simulink model "sampleModel334"  (R2021b)
settings: Solver=VariableStepAuto  StartTime=0.0  StopTime=10.0  RelTol=1e-3
undefined symbols (not defined in the file or in its folder): Newton, Raphson
libraries: simulink x13, slpidlib x2
settings Model: Creator=user  LastModifiedBy=user

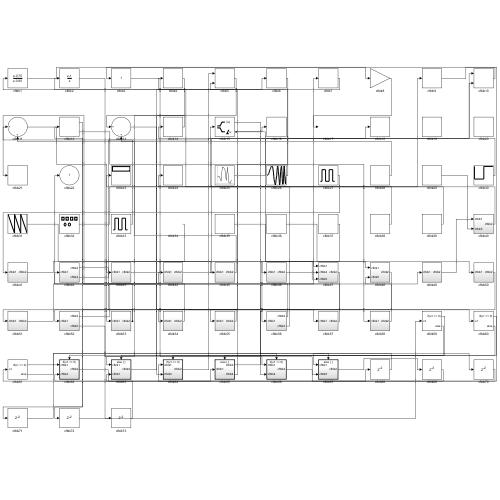
[thumbnail: Simulink's stored preview of the top-level diagram]
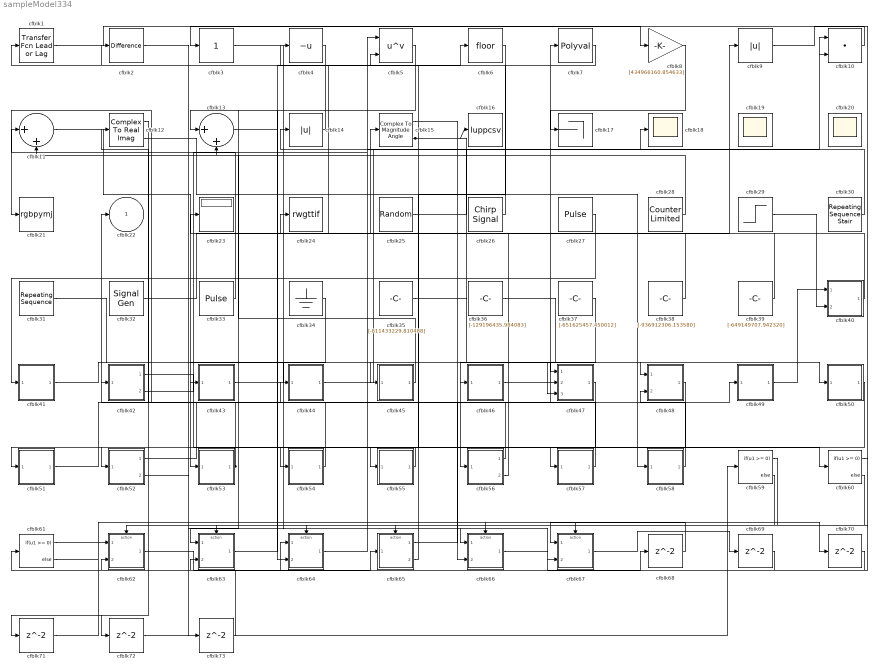
== system sampleModel334 ==
  cfblk1 : simulink/Discrete/Transfer Fcn Lead or Lag  PoleZ=0.95  ZeroZ=0.75  ICPrevOutput=0.0  ICPrevInput=0.0  DoSatur=off
      settings: SourceProductBaseCode=SL
  cfblk10 : DotProduct  InputSameDT=on  OutDataTypeStr=Inherit: Inherit via internal rule
  cfblk11 : Sum  Inputs=|++
  cfblk12 : ComplexToRealImag
  cfblk13 : Sum  Inputs=|++
  cfblk14 : Abs
  cfblk15 : ComplexToMagnitudeAngle
  cfblk16 : ToWorkspace  VariableName=luppcsv  SaveFormat=Timeseries  SampleTime=-1
  cfblk17 : Terminator
  cfblk18 : Scope
  cfblk19 : Scope
      settings: Floating=on
  cfblk2 : simulink/Discrete/Difference  ICPrevInput=0.0  OutMin=[]  OutMax=[]  OutDataTypeStr=Inherit: Inherit via back propagation  OutDataType=fixdt(1, 16)  OutScaling=2^-10  DoSatur=off
  cfblk20 : Scope
      settings: Floating=on
  cfblk21 : ToWorkspace  VariableName=rgbpymj  SaveFormat=Timeseries  SampleTime=-1
  cfblk23 : Display
  cfblk24 : ToWorkspace  VariableName=rwgttif  SaveFormat=Timeseries  SampleTime=-1
  cfblk25 : RandomNumber  Mean=[-31709.471709]  Variance=[21880.294975]  Seed=[988417570.000000]  SampleTime=0.1
  cfblk26 : simulink/Sources/Chirp Signal  f1=[-190654056.309968]  T=[-437298929.840146]  f2=[-613895744.060993]
  cfblk27 : DiscretePulseGenerator  PulseType=Time based  Amplitude=[95953160.588672]  Period=[92796952.421330]  PulseWidth=5  PhaseDelay=[6.000000]
  cfblk28 : simulink/Sources/Counter Limited  uplimit=[666.000000]  tsamp=-1
  cfblk29 : Step  Time=[43.000000]  Before=[594714500.417629]  After=[-95569825.791447]  SampleTime=0
  cfblk3 : simulink/Math Operations/Slider Gain  gain=1  low=0  high=2
  cfblk30 : simulink/Sources/Repeating Sequence Stair  OutValues=[445695939.025532, 871780423.496067]  tsamp=-1  OutMin=[]  OutMax=[]  OutDataTypeStr=double  OutputDataTypeScalingMode=double  OutDataType=fixdt(0,8)  ConRadixGroup=Best Precision: Vector-wise  OutScaling=2^-12
  cfblk31 : simulink/Sources/Repeating Sequence  rep_seq_t=[0 2]  rep_seq_y=[950228293.664763, -742331251.435693]
  cfblk32 : SignalGenerator  WaveForm=square  Amplitude=[-929706620.397252]
  cfblk33 : DiscretePulseGenerator  PulseType=Time based  Amplitude=[171272689.061584]  Period=[21777336.643876]  PulseWidth=5  PhaseDelay=[4.000000]
  cfblk34 : Ground
  cfblk35 : Constant  Value=[-811433229.810488]  SampleTime=1
  cfblk36 : Constant  Value=[-129196435.984083]  SampleTime=1
  cfblk37 : Constant  Value=[-651625457.450012]  SampleTime=1
  cfblk38 : Constant  Value=[-936912306.153580]  SampleTime=1
  cfblk39 : Constant  Value=[-649149707.942320]  SampleTime=1
  cfblk4 : UnaryMinus
  cfblk40 : Subsystem
  cfblk41 : Subsystem
  cfblk42 : Subsystem
  cfblk43 : Subsystem
  cfblk44 : Subsystem
  cfblk45 : Subsystem
  cfblk46 : Subsystem
  cfblk47 : Subsystem
  cfblk48 : Subsystem
  cfblk49 : Subsystem
  cfblk5 : Math  Operator=pow  SaturateOnIntegerOverflow=on
  cfblk50 : Subsystem
  cfblk51 : Subsystem
  cfblk52 : Subsystem
  cfblk53 : Subsystem
  cfblk54 : Subsystem
  cfblk55 : Subsystem
  cfblk56 : Subsystem
  cfblk57 : Subsystem
  cfblk58 : Subsystem
  cfblk59 : If  IfExpression=u1 >= 0  SampleTime=1
  cfblk6 : Rounding
  cfblk60 : If  IfExpression=u1 >= 0  SampleTime=1
  cfblk61 : If  IfExpression=u1 >= 0  SampleTime=1
  cfblk62 : Subsystem  TreatAsAtomicUnit=on
  cfblk63 : Subsystem  TreatAsAtomicUnit=on
  cfblk64 : Subsystem  TreatAsAtomicUnit=on
  cfblk65 : Subsystem  TreatAsAtomicUnit=on
  cfblk66 : Subsystem  TreatAsAtomicUnit=on
  cfblk67 : Subsystem  TreatAsAtomicUnit=on
  cfblk{68..73} (6 alike) : Delay  SampleTime=1
  cfblk7 : Polyval  Coefs=[ +2.081618890e-019, -1.441693666e-014, +4.719686976e-010, -8.536869453e-006, +1.621573104e-001, -8.087801117e+001 ]
  cfblk8 : Gain  Gain=[434966160.854633]
  cfblk9 : Abs
  cfblk22 : Outport
  wires:
  cfblk25/1 -> cfblk10/1
  cfblk14/1 -> cfblk13/1
  cfblk40/1(cfblk2) -> cfblk15/1
  cfblk49/1(cfblk2) -> cfblk40/1(cfblk1)
  cfblk57/1(cfblk2) -> cfblk21/1
  cfblk56/1(cfblk2) -> cfblk22/1
  cfblk43/1(cfblk2) -> cfblk48/1(cfblk1)
  cfblk37/1 -> cfblk56/1(cfblk1)
  cfblk3/1 -> cfblk66/1(cfblk1)
  cfblk30/1 -> cfblk14/1
  cfblk44/1(cfblk2) -> cfblk10/2
  cfblk33/1 -> cfblk11/1
  cfblk53/1(cfblk2) -> cfblk42/1(cfblk1), cfblk51/1(cfblk1)
  cfblk55/1(cfblk2) -> cfblk52/1(cfblk1)
  cfblk13/1 -> cfblk60/1
  cfblk12/2 -> cfblk58/1(cfblk1)
  cfblk31/1 -> cfblk46/1(cfblk1)
  cfblk51/1(cfblk2) -> cfblk44/1(cfblk1)
  cfblk27/1 -> cfblk41/1(cfblk1)
  cfblk1/1 -> cfblk8/1
  cfblk56/2(cfblk3) -> cfblk24/1
  cfblk42/1(cfblk2) -> cfblk57/1(cfblk1)
  cfblk42/2(cfblk4) -> cfblk5/1
  cfblk9/1 -> cfblk64/1(cfblk1)
  cfblk11/1 -> cfblk53/1(cfblk1)
  cfblk32/1 -> cfblk9/1
  cfblk36/1 -> cfblk50/1(cfblk1)
  cfblk7/1 -> cfblk5/2
  cfblk46/1(cfblk2) -> cfblk7/1
  cfblk58/1(cfblk2) -> cfblk48/2(cfblk5)
  cfblk28/1 -> cfblk11/2
  cfblk5/1 -> cfblk63/1(cfblk1)
  cfblk47/1(cfblk2) -> cfblk54/1(cfblk1)
  cfblk8/1 -> cfblk17/1
  cfblk10/1 -> cfblk3/1
  cfblk41/1(cfblk2) -> cfblk45/1(cfblk1)
  cfblk52/1(cfblk2) -> cfblk49/1(cfblk1)
  cfblk54/1(cfblk2) -> cfblk12/1
  cfblk34/1 -> cfblk43/1(cfblk1)
  cfblk2/1 -> cfblk67/2(cfblk5)
  cfblk62/1(cfblk2) -> cfblk65/1(cfblk1)
  cfblk4/1 -> cfblk64/2(cfblk3)
  cfblk45/1(cfblk2) -> cfblk13/2
  cfblk64/1(cfblk2) -> cfblk18/1
  cfblk15/2 -> cfblk16/1, cfblk47/3(cfblk5)
  cfblk6/1 -> cfblk55/1(cfblk1)
  cfblk26/1 -> cfblk2/1
  cfblk50/1(cfblk2) -> cfblk66/2(cfblk4)
  cfblk35/1 -> cfblk47/1(cfblk1)
  cfblk29/1 -> cfblk40/2(cfblk5)
  cfblk38/1 -> cfblk4/1
  cfblk63/1(cfblk2) -> cfblk6/1
  cfblk39/1 -> cfblk23/1
  cfblk65/1(cfblk2) -> cfblk47/2(cfblk4)
  cfblk65/2(cfblk4) -> cfblk1/1
  cfblk59/1 -> cfblk62/Action
  cfblk59/2 -> cfblk63/Action
  cfblk60/1 -> cfblk64/Action
  cfblk60/2 -> cfblk65/Action
  cfblk61/1 -> cfblk66/Action
  cfblk61/2 -> cfblk67/Action
  cfblk66/1(cfblk2) -> cfblk68/1
  cfblk68/1 -> cfblk67/1(cfblk1)
  cfblk67/1(cfblk2) -> cfblk69/1
  cfblk69/1 -> cfblk61/1
  cfblk15/1 -> cfblk70/1
  cfblk70/1 -> cfblk62/2(cfblk4)
  cfblk12/1 -> cfblk71/1
  cfblk71/1 -> cfblk62/1(cfblk1)
  cfblk48/1(cfblk2) -> cfblk72/1
  cfblk72/1 -> cfblk59/1
  cfblk52/2(cfblk5) -> cfblk73/1
  cfblk73/1 -> cfblk63/2(cfblk3)

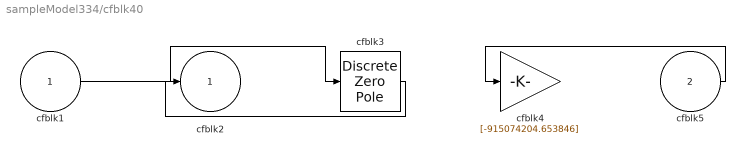
== system sampleModel334/cfblk40 ==
  cfblk1 : Inport
  cfblk5 : Inport  Port=2
  cfblk3 : DiscreteZeroPole  Poles=[0 0.5]  Gain=1
  cfblk4 : Gain  Gain=[-915074204.653846]
  cfblk2 : Outport
  wires:
  cfblk1/1 -> cfblk3/1
  cfblk3/1 -> cfblk2/1
  cfblk5/1 -> cfblk4/1

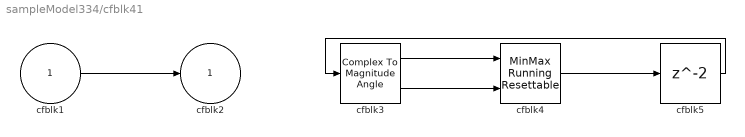
== system sampleModel334/cfblk41 ==
  cfblk1 : Inport
  cfblk3 : ComplexToMagnitudeAngle
  cfblk4 : simulink/Math Operations/MinMax Running Resettable  Function=min  vinit=0.0
  cfblk5 : Delay  SampleTime=1
  cfblk2 : Outport
  wires:
  cfblk1/1 -> cfblk2/1
  cfblk3/1 -> cfblk4/1
  cfblk3/2 -> cfblk4/2
  cfblk4/1 -> cfblk5/1
  cfblk5/1 -> cfblk3/1

== system sampleModel334/cfblk42 ==
  cfblk1 : Inport
  cfblk3 : Constant  Value=[-435309913.935289]  SampleTime=1
  cfblk2 : Outport
  cfblk4 : Outport  Port=2
  wires:
  cfblk3/1 -> cfblk2/1
  cfblk1/1 -> cfblk4/1

== system sampleModel334/cfblk43 ==
  cfblk1 : Inport
  cfblk3 : simulink/Math Operations/MinMax Running Resettable  Function=min  vinit=0.0
  cfblk4 : simulink/Math Operations/Slider Gain  gain=1  low=0  high=2
  cfblk2 : Outport
  wires:
  cfblk1/1 -> cfblk4/1
  cfblk4/1 -> cfblk3/1, cfblk3/2
  cfblk3/1 -> cfblk2/1

== system sampleModel334/cfblk44 ==
  cfblk1 : Inport
  cfblk3 : Product  Inputs=**
  cfblk2 : Outport
  wires:
  cfblk1/1 -> cfblk3/1, cfblk3/2
  cfblk3/1 -> cfblk2/1

== system sampleModel334/cfblk45 ==
  cfblk1 : Inport
  cfblk3 : DiscreteTransferFcn  SampleTime=1
  cfblk2 : Outport
  wires:
  cfblk1/1 -> cfblk3/1
  cfblk3/1 -> cfblk2/1

== system sampleModel334/cfblk46 ==
  cfblk1 : Inport
  cfblk3 : Abs
  cfblk2 : Outport
  wires:
  cfblk1/1 -> cfblk2/1, cfblk3/1

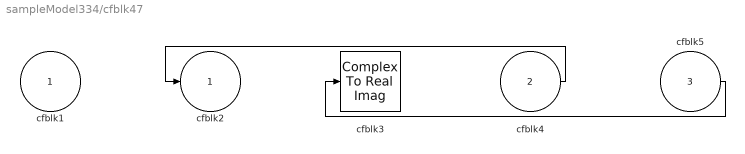
== system sampleModel334/cfblk47 ==
  cfblk1 : Inport
  cfblk4 : Inport  Port=2
  cfblk5 : Inport  Port=3
  cfblk3 : ComplexToRealImag
  cfblk2 : Outport
  wires:
  cfblk4/1 -> cfblk2/1
  cfblk5/1 -> cfblk3/1

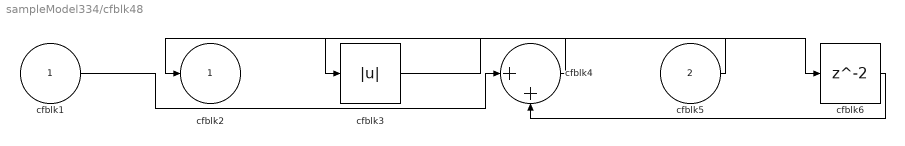
== system sampleModel334/cfblk48 ==
  cfblk1 : Inport
  cfblk5 : Inport  Port=2
  cfblk3 : Abs
  cfblk4 : Sum  Inputs=|++
  cfblk6 : Delay  SampleTime=1
  cfblk2 : Outport
  wires:
  cfblk5/1 -> cfblk2/1
  cfblk1/1 -> cfblk4/1
  cfblk4/1 -> cfblk3/1
  cfblk3/1 -> cfblk6/1
  cfblk6/1 -> cfblk4/2

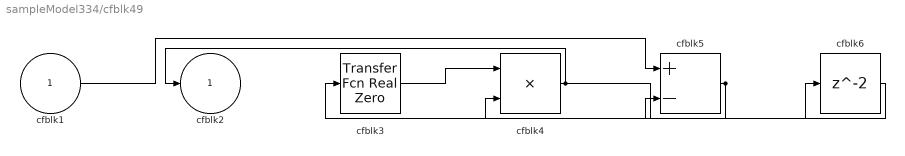
== system sampleModel334/cfblk49 ==
  cfblk1 : Inport
  cfblk3 : simulink/Discrete/Transfer Fcn Real Zero  ZeroZ=0.75  ICPrevInput=0.0  DoSatur=off
      settings: SourceProductBaseCode=SL
  cfblk4 : Product  Inputs=**
  cfblk5 : Sum  Inputs=+-
  cfblk6 : Delay  SampleTime=1
  cfblk2 : Outport
  wires:
  cfblk3/1 -> cfblk4/1
  cfblk4/1 -> cfblk2/1, cfblk6/1
  cfblk5/1 -> cfblk3/1, cfblk4/2
  cfblk1/1 -> cfblk5/1
  cfblk6/1 -> cfblk5/2

== system sampleModel334/cfblk50 ==
  cfblk1 : Inport
  cfblk3 : simulink/Math Operations/Slider Gain  gain=1  low=0  high=2
  cfblk2 : Outport
  wires:
  cfblk3/1 -> cfblk2/1
  cfblk1/1 -> cfblk3/1

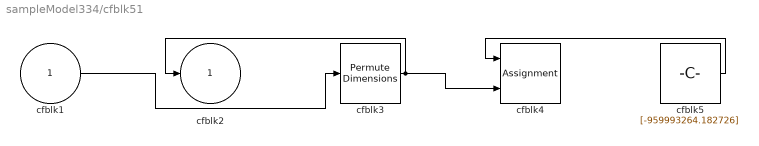
== system sampleModel334/cfblk51 ==
  cfblk1 : Inport
  cfblk3 : PermuteDimensions
  cfblk4 : Assignment  DiagnosticForDimensions=Warning  IndexOptions=Index vector (dialog)  Indices=1  OutputSizes=1
  cfblk5 : Constant  Value=[-959993264.182726]  SampleTime=1
  cfblk2 : Outport
  wires:
  cfblk3/1 -> cfblk2/1, cfblk4/2
  cfblk5/1 -> cfblk4/1
  cfblk1/1 -> cfblk3/1

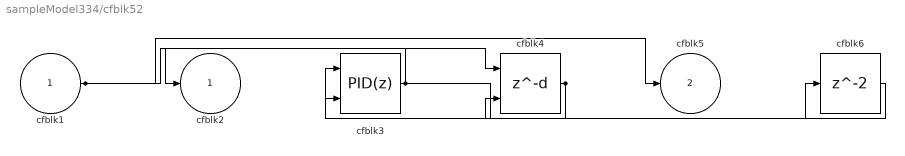
== system sampleModel334/cfblk52 ==
  cfblk1 : Inport
  cfblk3 : slpidlib/PID Controller (2DOF)  Controller=PID  Form=Parallel  TimeDomain=Discrete-time  UseExternalTs=off  SampleTime=1  IntegratorMethod=Forward Euler  FilterMethod=Forward Euler  ControllerParametersSource=internal  P=1  I=1  D=0  UseFilter=on  N=100  b=1  c=1  TunerSelectOption=Transfer Function Based (PID Tuner App)  InitialConditionSource=internal  InitialConditionForIntegrator=0  InitialConditionForFilter=0  DifferentiatorICPrevScaledInput=0  ExternalReset=none  TrackingMode=off  Kt=1  LimitOutput=off  SatLimitsSource=internal  UpperSaturationLimit=inf  LowerSaturationLimit=-inf  LinearizeAsGain=off  AntiWindupMode=none  Kb=1  POutMin=[]  POutMax=[]  IOutMin=[]  IOutMax=[]  DOutMin=[]  DOutMax=[]  NOutMin=[]  NOutMax=[]  bOutMin=[]  bOutMax=[]  cOutMin=[]  cOutMax=[]  SumOutMin=[]  SumOutMax=[]  SaturationOutMin=[]  SaturationOutMax=[]  PParamMin=[]  PParamMax=[]  IParamMin=[]  IParamMax=[]  DParamMin=[]  DParamMax=[]  NParamMin=[]  NParamMax=[]  bParamMin=[]  bParamMax=[]  cParamMin=[]  cParamMax=[]  KbParamMin=[]  KbParamMax=[]  KtParamMin=[]  KtParamMax=[]  KbOutMin=[]  KbOutMax=[]  KtOutMin=[]  KtOutMax=[]  IntegratorOutMin=[]  IntegratorOutMax=[]  FilterOutMin=[]  FilterOutMax=[]  SumI1OutMin=[]  SumI1OutMax=[]  SumI2OutMin=[]  SumI2OutMax=[]  SumI3OutMin=[]  SumI3OutMax=[]  SumI4OutMin=[]  SumI4OutMax=[]  SumDOutMin=[]  SumDOutMax=[]  Sum1OutMin=[]  Sum1OutMax=[]  Sum2OutMin=[]  Sum2OutMax=[]  Sum3OutMin=[]  Sum3OutMax=[]  DifferentiatorOutMin=[]  DifferentiatorOutMax=[]  FilterDiffOutCoefMin=[]  FilterDiffOutCoefMax=[]  ReciprocalOutMin=[]  ReciprocalOutMax=[]  SumDenOutMin=[]  SumDenOutMax=[]  SumNumOutMin=[]  SumNumOutMax=[]  DivideOutMin=[]  DivideOutMax=[]  UdiffTsProdOutMin=[]  UdiffTsProdOutMax=[]  NTsProdOutMin=[]  NTsProdOutMax=[]  UintegralTsProdOutMin=[]  UintegralTsProdOutMax=[]  UngainTsProdOutMin=[]  UngainTsProdOutMax=[]  IntegratorContinuousStateAttributes=''  IntegratorStateMustResolveToSignalObject=off  IntegratorRTWStateStorageClass=Auto  FilterContinuousStateAttributes=''  FilterStateMustResolveToSignalObject=off  FilterRTWStateStorageClass=Auto  ParallelPVariant=InternalParameters  IdealPVariant=Disabled  IVariant=InternalParameters  DVariant=InternalParameters  bVariant=InternalParameters  cVariant=InternalParameters  IntegratorVariant=Discrete  SatVariant=Disabled  AWVariant=Passthrough  PCopyVariant=Disabled  TRVariant=Disabled  FdbkBlocksVariant=Forward  IdealPFdbkVariant=Disabled  SatFdbkVariant=Disabled  DerivativeFilterVariant=ForwardEulerFilter  NVariant=InternalParameters  NCopyVariant=Disabled  FilterICVariant=InternalICsFilter  IntegratorICVariant=InternalICs  ExternalResetVariant=Disabled  TRSumVariant=Passthrough  SumFdbkVariant=Disabled  SumVariant=Sum_PID  TsampFilterVariant=InternalTs  TsampNgainVariant=Passthrough  TsampIntegralVariant=Passthrough  ExternalSaturationOutDataTypeStr=Inherit: Same as second input
      settings: SourceProductBaseCode=SL
  cfblk4 : Delay  DelayLengthSource=Input port  SampleTime=1
      settings: InputPortMap=u0,p1
  cfblk6 : Delay  SampleTime=1
  cfblk2 : Outport
  cfblk5 : Outport  Port=2
  wires:
  cfblk3/1 -> cfblk2/1, cfblk6/1
  cfblk4/1 -> cfblk3/1, cfblk3/2
  cfblk1/1 -> cfblk5/1, cfblk4/1
  cfblk6/1 -> cfblk4/2

== system sampleModel334/cfblk53 ==
  cfblk1 : Inport
  cfblk3 : slpidlib/PID Controller (2DOF)  Controller=PID  Form=Parallel  TimeDomain=Discrete-time  UseExternalTs=off  SampleTime=1  IntegratorMethod=Forward Euler  FilterMethod=Forward Euler  ControllerParametersSource=internal  P=1  I=1  D=0  UseFilter=on  N=100  b=1  c=1  TunerSelectOption=Transfer Function Based (PID Tuner App)  InitialConditionSource=internal  InitialConditionForIntegrator=0  InitialConditionForFilter=0  DifferentiatorICPrevScaledInput=0  ExternalReset=none  TrackingMode=off  Kt=1  LimitOutput=off  SatLimitsSource=internal  UpperSaturationLimit=inf  LowerSaturationLimit=-inf  LinearizeAsGain=off  AntiWindupMode=none  Kb=1  POutMin=[]  POutMax=[]  IOutMin=[]  IOutMax=[]  DOutMin=[]  DOutMax=[]  NOutMin=[]  NOutMax=[]  bOutMin=[]  bOutMax=[]  cOutMin=[]  cOutMax=[]  SumOutMin=[]  SumOutMax=[]  SaturationOutMin=[]  SaturationOutMax=[]  PParamMin=[]  PParamMax=[]  IParamMin=[]  IParamMax=[]  DParamMin=[]  DParamMax=[]  NParamMin=[]  NParamMax=[]  bParamMin=[]  bParamMax=[]  cParamMin=[]  cParamMax=[]  KbParamMin=[]  KbParamMax=[]  KtParamMin=[]  KtParamMax=[]  KbOutMin=[]  KbOutMax=[]  KtOutMin=[]  KtOutMax=[]  IntegratorOutMin=[]  IntegratorOutMax=[]  FilterOutMin=[]  FilterOutMax=[]  SumI1OutMin=[]  SumI1OutMax=[]  SumI2OutMin=[]  SumI2OutMax=[]  SumI3OutMin=[]  SumI3OutMax=[]  SumI4OutMin=[]  SumI4OutMax=[]  SumDOutMin=[]  SumDOutMax=[]  Sum1OutMin=[]  Sum1OutMax=[]  Sum2OutMin=[]  Sum2OutMax=[]  Sum3OutMin=[]  Sum3OutMax=[]  DifferentiatorOutMin=[]  DifferentiatorOutMax=[]  FilterDiffOutCoefMin=[]  FilterDiffOutCoefMax=[]  ReciprocalOutMin=[]  ReciprocalOutMax=[]  SumDenOutMin=[]  SumDenOutMax=[]  SumNumOutMin=[]  SumNumOutMax=[]  DivideOutMin=[]  DivideOutMax=[]  UdiffTsProdOutMin=[]  UdiffTsProdOutMax=[]  NTsProdOutMin=[]  NTsProdOutMax=[]  UintegralTsProdOutMin=[]  UintegralTsProdOutMax=[]  UngainTsProdOutMin=[]  UngainTsProdOutMax=[]  IntegratorContinuousStateAttributes=''  IntegratorStateMustResolveToSignalObject=off  IntegratorRTWStateStorageClass=Auto  FilterContinuousStateAttributes=''  FilterStateMustResolveToSignalObject=off  FilterRTWStateStorageClass=Auto  ParallelPVariant=InternalParameters  IdealPVariant=Disabled  IVariant=InternalParameters  DVariant=InternalParameters  bVariant=InternalParameters  cVariant=InternalParameters  IntegratorVariant=Discrete  SatVariant=Disabled  AWVariant=Passthrough  PCopyVariant=Disabled  TRVariant=Disabled  FdbkBlocksVariant=Forward  IdealPFdbkVariant=Disabled  SatFdbkVariant=Disabled  DerivativeFilterVariant=ForwardEulerFilter  NVariant=InternalParameters  NCopyVariant=Disabled  FilterICVariant=InternalICsFilter  IntegratorICVariant=InternalICs  ExternalResetVariant=Disabled  TRSumVariant=Passthrough  SumFdbkVariant=Disabled  SumVariant=Sum_PID  TsampFilterVariant=InternalTs  TsampNgainVariant=Passthrough  TsampIntegralVariant=Passthrough  ExternalSaturationOutDataTypeStr=Inherit: Same as second input
      settings: SourceProductBaseCode=SL
  cfblk2 : Outport
  wires:
  cfblk3/1 -> cfblk2/1
  cfblk1/1 -> cfblk3/1, cfblk3/2

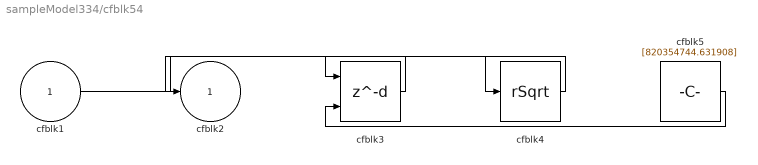
== system sampleModel334/cfblk54 ==
  cfblk1 : Inport
  cfblk3 : Delay  DelayLengthSource=Input port  SampleTime=1
      settings: InputPortMap=u0,p1
  cfblk4 : Sqrt  Operator=rSqrt  AlgorithmType=Newton-Raphson  SaturateOnIntegerOverflow=on
  cfblk5 : Constant  Value=[820354744.631908]  SampleTime=1
  cfblk2 : Outport
  wires:
  cfblk4/1 -> cfblk3/1
  cfblk5/1 -> cfblk3/2
  cfblk1/1 -> cfblk4/1
  cfblk3/1 -> cfblk2/1

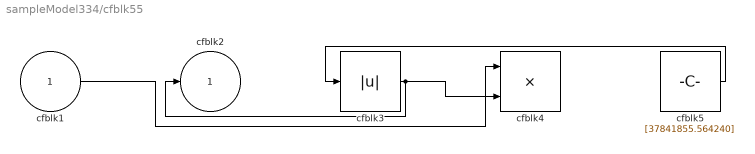
== system sampleModel334/cfblk55 ==
  cfblk1 : Inport
  cfblk3 : Abs
  cfblk4 : Product  Inputs=**
  cfblk5 : Constant  Value=[37841855.564240]  SampleTime=1
  cfblk2 : Outport
  wires:
  cfblk5/1 -> cfblk3/1
  cfblk3/1 -> cfblk2/1, cfblk4/2
  cfblk1/1 -> cfblk4/1

== system sampleModel334/cfblk56 ==
  cfblk1 : Inport
  cfblk2 : Outport
  cfblk3 : Outport  Port=2
  wires:
  cfblk1/1 -> cfblk2/1, cfblk3/1

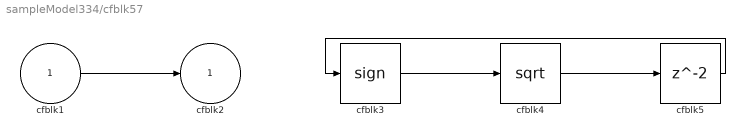
== system sampleModel334/cfblk57 ==
  cfblk1 : Inport
  cfblk3 : Signum
  cfblk4 : Sqrt  SaturateOnIntegerOverflow=on
  cfblk5 : Delay  SampleTime=1
  cfblk2 : Outport
  wires:
  cfblk1/1 -> cfblk2/1
  cfblk3/1 -> cfblk4/1
  cfblk4/1 -> cfblk5/1
  cfblk5/1 -> cfblk3/1

== system sampleModel334/cfblk58 ==
  cfblk1 : Inport
  cfblk3 : Reshape
  cfblk4 : Sum
  cfblk2 : Outport
  wires:
  cfblk3/1 -> cfblk4/1
  cfblk1/1 -> cfblk4/2, cfblk3/1
  cfblk4/1 -> cfblk2/1

== system sampleModel334/cfblk62 ==
  cfblk1 : Inport
  cfblk4 : Inport  Port=2
  Action Port : ActionPort  ActionPortLabel=if(u1 >= 0)
  cfblk3 : Abs
  cfblk2 : Outport
  wires:
  cfblk4/1 -> cfblk3/1
  cfblk1/1 -> cfblk2/1

== system sampleModel334/cfblk63 ==
  cfblk1 : Inport
  cfblk3 : Inport  Port=2
  Action Port : ActionPort  ActionPortLabel=else
  cfblk2 : Outport
  wires:
  cfblk1/1 -> cfblk2/1

== system sampleModel334/cfblk64 ==
  cfblk1 : Inport
  cfblk3 : Inport  Port=2
  Action Port : ActionPort  ActionPortLabel=if(u1 >= 0)
  cfblk2 : Outport
  wires:
  cfblk1/1 -> cfblk2/1

== system sampleModel334/cfblk65 ==
  cfblk1 : Inport
  Action Port : ActionPort  ActionPortLabel=else
  cfblk3 : simulink/Discrete/Tapped Delay  vinit=0.0  samptime=-1  NumDelays=1  DelayOrder=Oldest  includeCurrent=off
  cfblk2 : Outport
  cfblk4 : Outport  Port=2
  wires:
  cfblk1/1 -> cfblk4/1, cfblk3/1
  cfblk3/1 -> cfblk2/1

== system sampleModel334/cfblk66 ==
  cfblk1 : Inport
  cfblk4 : Inport  Port=2
  Action Port : ActionPort  ActionPortLabel=if(u1 >= 0)
  cfblk3 : Sin  TimeSource=Use external signal  SampleTime=0
  cfblk2 : Outport
  wires:
  cfblk4/1 -> cfblk2/1
  cfblk1/1 -> cfblk3/1

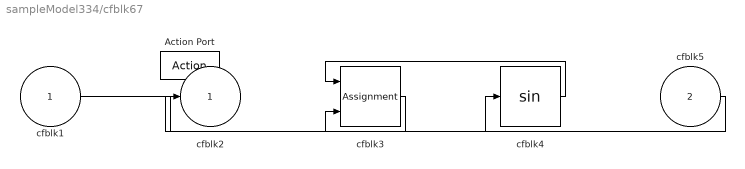
== system sampleModel334/cfblk67 ==
  cfblk1 : Inport
  cfblk5 : Inport  Port=2
  Action Port : ActionPort  ActionPortLabel=else
  cfblk3 : Assignment  DiagnosticForDimensions=Warning  IndexOptions=Index vector (dialog)  Indices=1  OutputSizes=1
  cfblk4 : Trigonometry
  cfblk2 : Outport
  wires:
  cfblk4/1 -> cfblk3/1
  cfblk5/1 -> cfblk3/2
  cfblk1/1 -> cfblk4/1
  cfblk3/1 -> cfblk2/1
